simulink library "simple_mosfet"  (R2025b)
settings: Solver=VariableStepAuto  StartTime=0.0  StopTime=10.0  RelTol=1e-3
undefined symbols (not defined in the file): mosfet
libraries: nesl_utility x2, basic_mosfet_lib x1, fl_lib x1
settings Model: Creator=dbagn  LastModifiedBy=dbagn

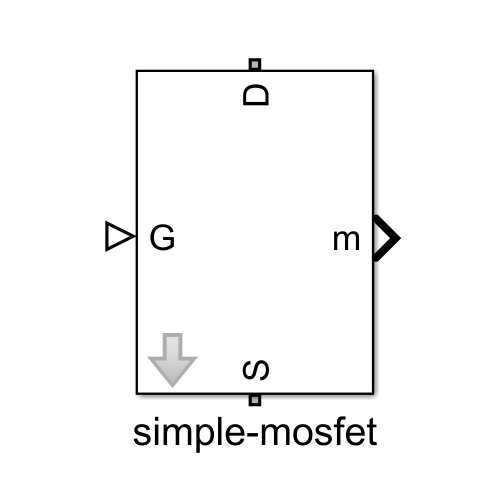
[thumbnail: Simulink's stored preview of the top-level diagram]
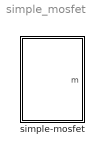
== system simple_mosfet ==
  simple-mosfet : Subsystem  mask{Rds_on_m=mosfet.inv.Rds_on, Vth_m=mosfet.inv.Vth, g_fs_m=mosfet.inv.g_fs, Vdon_diode_m=mosfet.inv.Vdon_diode, Rdon_diode_m=mosfet.inv.Rdon_diode}
      mask prompts: Rds_on_m "Rds_on (Ohm)"; Vth_m "Vth (V)"; g_fs_m "g_fs (A/V)"; Vdon_diode_m "Vdon_diode (V)"; Rdon_diode_m "Rdon_diode (Ohm)"
      settings: PortSchema="{\"entries\":[{\"content\":{\"sides\":[{\"content\":{\"connectorIds\":[\"LConn1\"]},\"type\":\"ConnectorPlacement.EquallySpacedRectSide\",\"uuid\":\"325dc963-858c-47f0-8995-f323ab4d9c46\"},{\"content\":{\"connectorIds\":[\"Out1\"],\"side\":\"RIGHT\"},\"type\":\"ConnectorPlacement.EquallySpacedRectSide\",\"uuid\":\"e9e66084-ecb2-40fb-9a1e-77677e0cc1df\"},{\"content\":{\"connectorIds\":[\"LConn2\"],\"side\":\"TOP\"},\"type\":\"ConnectorPlacement.EquallySpacedRectSide\",\"uuid\":\"9480d797-f2f6-459b-bb7c-d63861b57fde\"},{\"content\":{\"connectorIds\":[\"RConn1\"],\"side\":\"BOTTOM\"},\"type\":\"ConnectorPlacement.EquallySpacedRectSide\",\"uuid\":\"b13176d9-73b9-4822-9a0d-ec75065272bc\"}]},\"type\":\"ConnectorPlacement.EquallySpacedConnector\",\"uuid\":\"5e4a07d9-f5e8-4613-9049-5a866b5d2453\"}],\"packageUris\":[\"http://schema.mathworks.com/mf0/Connector/R2020b\"],\"version\":\"1.0\"}"

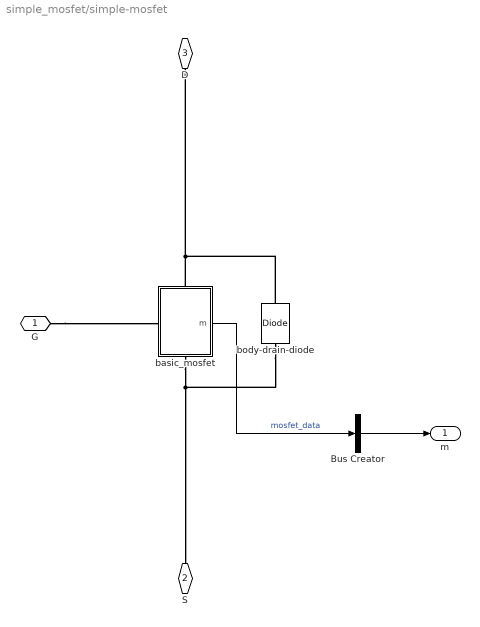
== system simple_mosfet/simple-mosfet ==
  Bus Creator : BusCreator  Inputs=1
  basic_mosfet : Subsystem  mask{Vth_m=Vth_m, Rds_on_m=Rds_on_m, g_fs_m=g_fs_m}
      mask prompts: Vth_m "Vth (V)"; Rds_on_m "Rds_on (Ohm)"; g_fs_m "g_fs (A/V)"
      settings: PortSchema="{\"entries\":[{\"content\":{\"sides\":[{\"content\":{\"connectorIds\":[\"LConn1\"]},\"type\":\"ConnectorPlacement.EquallySpacedRectSide\",\"uuid\":\"325dc963-858c-47f0-8995-f323ab4d9c46\"},{\"content\":{\"connectorIds\":[\"Out1\"],\"side\":\"RIGHT\"},\"type\":\"ConnectorPlacement.EquallySpacedRectSide\",\"uuid\":\"e9e66084-ecb2-40fb-9a1e-77677e0cc1df\"},{\"content\":{\"connectorIds\":[\"LConn2\"],\"side\":\"TOP\"},\"type\":\"ConnectorPlacement.EquallySpacedRectSide\",\"uuid\":\"9480d797-f2f6-459b-bb7c-d63861b57fde\"},{\"content\":{\"connectorIds\":[\"RConn1\"],\"side\":\"BOTTOM\"},\"type\":\"ConnectorPlacement.EquallySpacedRectSide\",\"uuid\":\"bd6f7c3f-e73f-43a3-8bfd-bc4aa1f2c71d\"}]},\"type\":\"ConnectorPlacement.EquallySpacedConnector\",\"uuid\":\"5e4a07d9-f5e8-4613-9049-5a866b5d2453\"}],\"packageUris\":[\"http://schema.mathworks.com/mf0/Connector/R2020b\"],\"version\":\"1.0\"}"
  body-drain-diode : fl_lib/Electrical/Electrical Elements/Diode  Vf=Vdon_diode_m V  Ron=Rdon_diode_m Ohm  Goff=1e-8 1/Ohm  i_specify=off  i_priority=None  i=0 A  i_nominal_specify=off  i_nominal_value=1  i_nominal_unit=A  v_specify=off  v_priority=None  v=0 V  v_nominal_specify=off  v_nominal_value=1  v_nominal_unit=V
  G : PMIOPort  Side=Left
  S : PMIOPort  Port=2  Side=Left
  D : PMIOPort  Port=3  Side=Right
  m : Outport
  wires:
  Bus Creator/1 -> m/1
  basic_mosfet/1(m) -> Bus Creator/1  "mosfet_data"
  connections:
  basic_mosfet/RConn1 -- S/RConn1 -- body-drain-diode/LConn1
  basic_mosfet/LConn2 -- D/RConn1 -- body-drain-diode/RConn1
  G/RConn1 -- basic_mosfet/LConn1

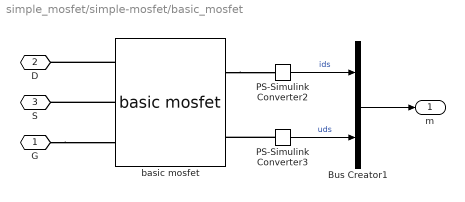
== system simple_mosfet/simple-mosfet/basic_mosfet ==
  Bus Creator1 : BusCreator  Inputs=2
  PS-Simulink Converter2 : nesl_utility/PS-Simulink Converter  PhysicalDomain=network_engine_domain  SubClassName=ps_output  LeftPortType=input  RightPortType=output  PseudoPeriodic=off  Frequencies=[]  VectorFormat=1-D array  Unit=A  AffineConversion=off
  PS-Simulink Converter3 : nesl_utility/PS-Simulink Converter  PhysicalDomain=network_engine_domain  SubClassName=ps_output  LeftPortType=input  RightPortType=output  PseudoPeriodic=off  Frequencies=[]  VectorFormat=1-D array  Unit=V  AffineConversion=off
  basic mosfet : basic_mosfet_lib/basic mosfet  Vth=Vth_m V  g_fs=g_fs_m A/V  Rds_on=Rds_on_m Ohm  ids_specify=off  ids_priority=High  ids=0 A  ids_nominal_specify=off  ids_nominal_value=1  ids_nominal_unit=A  uds_specify=off  uds_priority=None  uds=0 V  uds_nominal_specify=off  uds_nominal_value=1  uds_nominal_unit=V  ib_specify=off  ib_priority=None  ib=0 A  ib_nominal_specify=off  ib_nominal_value=1  ib_nominal_unit=A  ids_on_specify=off  ids_on_priority=None  ids_on=0 A  ids_on_nominal_specify=off  ids_on_nominal_value=1  ids_on_nominal_unit=A
      settings: InternalSimscapePortConfiguration="{\"Bottom\":[],\"Left\":[{\"id\":\"D\",\"label\":\"D\",\"type\":\"foundation.electrical.electrical\"},{\"id\":\"S\",\"label\":\"S\",\"type\":\"foundation.electrical.electrical\"},{\"id\":\"ugs\",\"label\":\"ugs\",\"type\":\"input\"}],\"Right\":[{\"id\":\"ids_out\",\"label\":\"ids\",\"type\":\"output\"},{\"id\":\"uds_out\",\"label\":\"uds\",\"type\":\"output\"}],\"Top\":[]}"
  G : PMIOPort  Side=Left
  D : PMIOPort  Port=2  Side=Left
  S : PMIOPort  Port=3  Side=Right
  m : Outport
  wires:
  PS-Simulink Converter3/1 -> Bus Creator1/2  "uds"
  PS-Simulink Converter2/1 -> Bus Creator1/1  "ids"
  Bus Creator1/1 -> m/1
  connections:
  basic mosfet/LConn2 -- S/RConn1
  basic mosfet/LConn1 -- D/RConn1
  basic mosfet/RConn1 -- PS-Simulink Converter2/LConn1
  PS-Simulink Converter3/LConn1 -- basic mosfet/RConn2
  G/RConn1 -- basic mosfet/LConn3
